simulink subsystem "boundary_subsys"  (R2025b)
settings: Solver=VariableStepAuto  StartTime=0.0  StopTime=10.0  RelTol=1e-3
undefined symbols (not defined in the file or in its folder): FL, WL
settings Model: Creator=Andrei  LastModifiedBy=Andrei

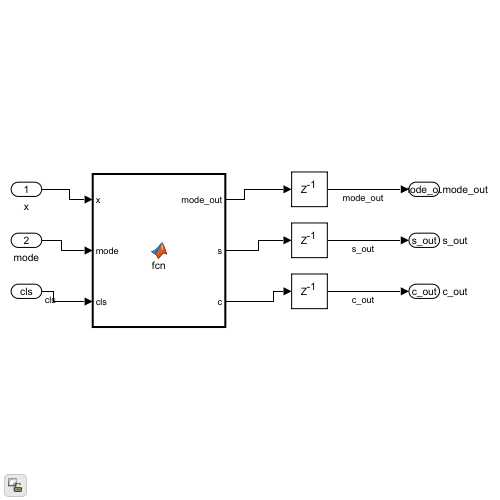
[thumbnail: Simulink's stored preview of the top-level diagram]
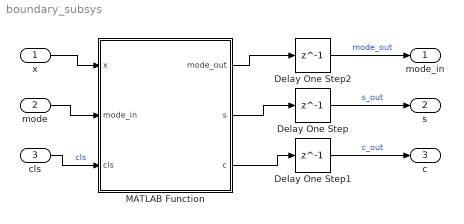
== system boundary_subsys ==
  x : Inport
  mode : Inport  Port=2
  cls : Inport  Port=3
  Delay One Step : Delay  DelayLength=1
  Delay One Step1 : Delay  DelayLength=1
  Delay One Step2 : Delay  DelayLength=1
  MATLAB Function : MATLAB Function  TreatAsAtomicUnit=on
  mode_in : Outport  SignalName=mode_out
  s : Outport  Port=2  SignalName=s_out
  c : Outport  Port=3  SignalName=c_out
  wires:
  MATLAB Function/1(mode_out) -> Delay One Step2/1
  x/1 -> MATLAB Function/1(x)
  cls/1 -> MATLAB Function/3(cls)  "cls"
  mode/1 -> MATLAB Function/2(mode_in)
  MATLAB Function/2(s) -> Delay One Step/1
  Delay One Step1/1 -> c/1  "c_out"
  Delay One Step/1 -> s/1  "s_out"
  MATLAB Function/3(c) -> Delay One Step1/1
  Delay One Step2/1 -> mode_in/1  "mode_out"

== matlab function boundary_subsys/MATLAB Function ==
  data: mode_out output; x input; s output; mode_in input; cls input; c output; WL parameter; FL parameter
function [mode_out, s,c]= fcn(x, mode_in, cls, WL, FL)

T = numerictype(1, WL, FL);
% T trebuie declarat în prealabil

persistent p_state;
if isempty(p_state)
    p_state = fi(0, 1, WL, FL);
end


s = fi(0, T);
c = fi(0, T);
mode_out = mode_in;

if cls
    p_state(:) = fi(0, 1, WL, FL);
    c = fi(0, 1, WL, FL);
    s = fi(0, 1, WL, FL);
else
    if mode_in == 1 % 1 - mode 1, 0 - mode 2 (așa a zis articolul)
        if abs(x) > abs(p_state)
            s = fi(1, 1, WL, FL);
            c(:) = -p_state/x;
            p_state(:) = x;
        else
            if p_state==0 % safe division, evităm cazul 0/0
                s=fi(0, 1, WL, FL);
                c=fi(0, 1, WL, FL);
            else
                s = fi(0, 1, WL, FL);
                c(:) = -x/p_state;
            end
        end
    else
        if p_state==0
            s=fi(0, 1, WL, FL);
            c=fi(0, 1, WL, FL);
        else
            s =fi(0, 1, WL, FL);
            c(:) = -x/p_state;
        end
    end
end
